simulink model "state_space"  (R2022b)
settings: Solver=VariableStepAuto  StartTime=0.0  StopTime=10.0  RelTol=1e-3
settings Model: Creator=hayden  LastModifiedBy=hayden

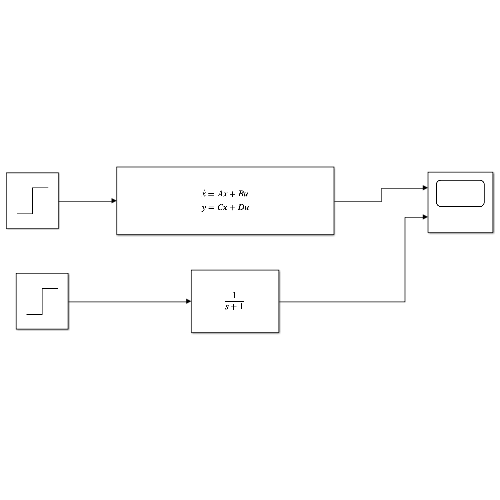
[thumbnail: Simulink's stored preview of the top-level diagram]
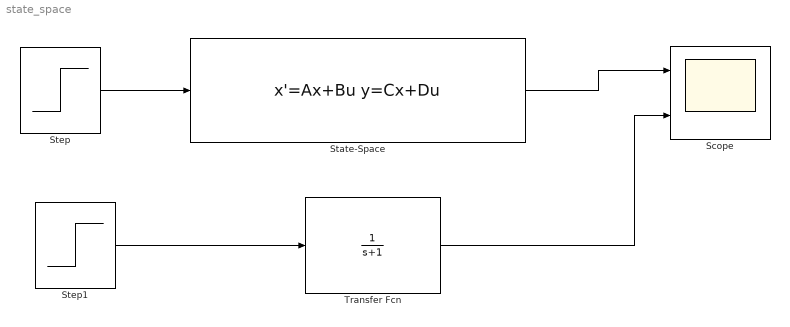
== system state_space ==
  Scope : Scope  NumInputPorts=2
  State-Space : StateSpace  A=-1  D=0  InitialCondition=0
  Step : Step  SampleTime=0
  Step1 : Step  Time=2  SampleTime=0
  Transfer Fcn : TransferFcn  Denominator=[1 1]
  wires:
  Step/1 -> State-Space/1
  State-Space/1 -> Scope/1
  Transfer Fcn/1 -> Scope/2
  Step1/1 -> Transfer Fcn/1
